simulink library "hcu_lib"  (Simulink 7.4)
settings: Solver=ode45  SolverMode=SingleTasking  StartTime=0.0  StopTime=10.0  RelTol=1e-3
undefined symbols (not defined in the file): FALSE, KPH2MPH, KPH2MPS, MPH2KPH, MPS2KPH, RADPS2RPM, RPM2RADPS, TRUE
libraries: hcu_lib x5, simulink x4
settings Model: Creator=gpf  LastModifiedBy=WX  ExtModeAutoUpdateStatusClock=off

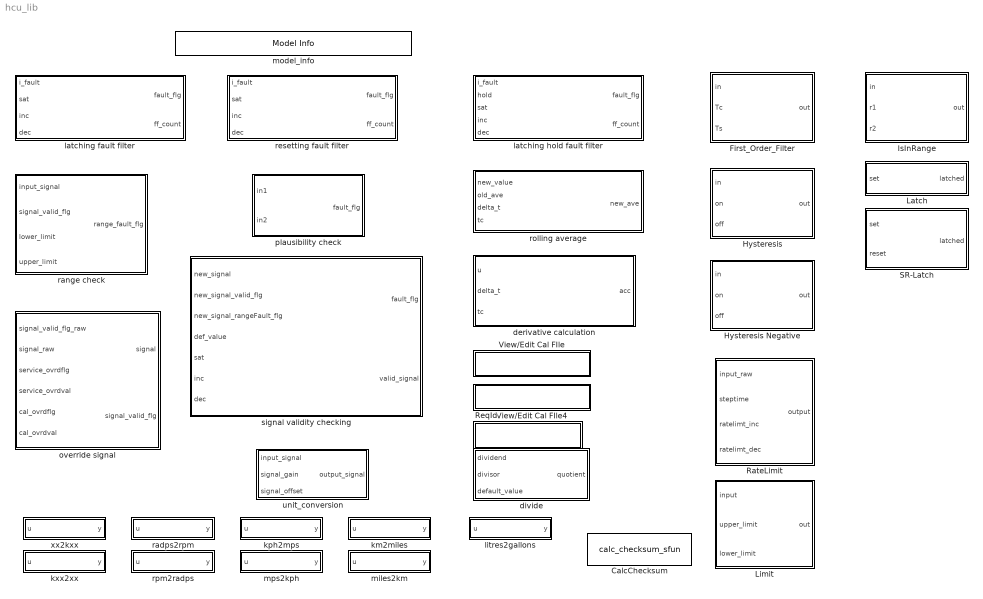
== system hcu_lib ==
  CalcChecksum : S-Function  FunctionName=calc_checksum_sfun  Parameters=seed_val  EnableBusSupport=off  mask(CalcChecksum){seed_val=40535}
      mask prompts: seed_val "seed (decimal)"
      mask help:
      | Sums the first 6 bytes on the input and returns a uint16 checksum value. The
      | input is a vector of 8 bytes (uint8).
      mask Display: fprintf('calc_checksum\nseed=%d',seed_val);
  First_Order_Filter : Subsystem  TreatAsAtomicUnit=on  RTWFileName=HCU_LIB
      settings: RTWFileNameOpts=User specified
  Hysteresis : Subsystem  TreatAsAtomicUnit=on  RTWFileName=HCU_LIB
      settings: RTWFileNameOpts=User specified
  Hysteresis Negative : Subsystem  TreatAsAtomicUnit=on  RTWFileName=HCU_LIB
      settings: RTWFileNameOpts=User specified
  IsInRange : Subsystem  TreatAsAtomicUnit=on  RTWFileName=HCU_LIB
      settings: RTWFileNameOpts=User specified
  Latch : Subsystem
  Limit : Subsystem  TreatAsAtomicUnit=on  RTWFileName=HCU_LIB
      settings: RTWFileNameOpts=User specified
  RateLimit : Subsystem  TreatAsAtomicUnit=on  RTWFileName=HCU_LIB
      settings: RTWFileNameOpts=User specified
  ReqId : Subsystem  mask(ReqId){req_str=HCU_000}
      mask prompts: req_str "Requirement:"
      mask help: Requirement Id
      mask Display: disp(sprintf('ReqId: %s',req_str));
  SR-Latch : Subsystem
  View/Edit Cal FIle : Subsystem  mask(edit){filename=foo}
      mask help:
      | Double-click to open the named file for viewing/editing.
      |
      | To set the name of the file opened, right-click on the block
      | and select Mask Parameters, and enter the name of the file,
      | which must be on the matlab path, without the .m extension.
      mask Help:
      | Double-click to open the named file for viewing/editing.
      | 
      | To set the name of the file opened, right-click on the block
      | and select Mask Parameters, and enter the name of the file,
      | which must be on the matlab path, without the .m extension.
      mask Display: disp(sprintf('Edit M-File: %s.m',filename));
  View/Edit Cal FIle4 : Subsystem  mask(run){filename=, run_on_load=off, run_on_init=off}
      mask prompts: run_on_load "run file on loading model"; run_on_init "run file on init"
      mask help:
      | Double-click to execute the named file.
      |
      | To set the name of the file, right-click on the block
      | and select Mask Parameters, and enter the name of the file,
      | which must be on the matlab path, without the .m extension.
      mask Help:
      | Double-click to execute the named file.
      | 
      | To set the name of the file, right-click on the block
      | and select Mask Parameters, and enter the name of the file,
      | which must be on the matlab path, without the .m extension.
      mask Display: disp(sprintf('Run M-File: %s.m',filename));
  derivative calculation : Subsystem  TreatAsAtomicUnit=on  RTWFileName=HCU_LIB  mask(Derative Block){lower_limit=, upper_limit=, time_const=}
      mask prompts: lower_limit "Lower Limit"; upper_limit "Upper Limit"; time_const "Time Constant"
      mask help: Derivative Calculation
      settings: RTWFileNameOpts=User specified
      mask Display: disp(['Derivative\nTC: ', get_param(gcb,'time_const'), '\nLower Limit: ', get_param(gcb, 'lower_limit'), '\nUpper Limit: ', get_param(gcb, 'upper_limit')])
  divide : Subsystem  TreatAsAtomicUnit=on  RTWFcnName=plaus_check
      settings: RTWSystemCode=Inline  RTWFcnNameOpts=User specified
      mask Type: divide
      mask Description: Performs a division operation. If the divisor is found to be between -0.00001 and +0.00001 then a failsafe value is passed to the output.
      mask Display: disp('Divide');
  km2miles : Subsystem
      mask Type: Conversion
      mask Description: Convert kilometers to miles.
      mask Display: disp('km \rightarrow mile', 'texmode', 'on')
  kph2mps : Subsystem
      mask Type: Conversion
      mask Description: Convert Kilometers per hour to Meters per second
      mask Display: disp('km/h \rightarrow m/s', 'texmode', 'on')
  kxx2xx : Subsystem
      mask Type: Conversion
      mask Description: Multiply by 1000.
      mask Display: disp('kiloxx \rightarrow xx', 'texmode', 'on')
  latching fault filter : Subsystem  TreatAsAtomicUnit=on  RTWFcnName=ff_latching  RTWFileName=HCU_LIB
      settings: RTWFcnNameOpts=User specified  RTWFileNameOpts=User specified
      mask Type: Latching Fault Filter
      mask Description: Fault filter block - Latches the fault output flag to TRUE if the input flag is repeatedly set True.
      mask Display: disp('Latching\nFault Filter')
  latching hold fault filter : Subsystem  TreatAsAtomicUnit=on  RTWFcnName=ff_latchhold  RTWFileName=HCU_LIB  mask(Latching Holdable Fault Filter){inc=, dec=, sat=}
      mask prompts: inc "increment"; dec "decrement"; sat "limit"
      mask help: Fault Filter Block - Latches output flag once set. Also fault count can be held at a value if the hold input is set.
      settings: RTWFcnNameOpts=User specified  RTWFileNameOpts=User specified
      mask Display: disp('Latching Holdable\nFault Filter')
  litres2gallons : Subsystem  mask(Conversion){UK=off}
      mask prompts: UK "UK Gallon"
      mask help: Convert litres to gallons.
      mask Display: disp('litre \rightarrow gallon', 'texmode', 'on')
  miles2km : Subsystem
      mask Type: Conversion
      mask Description: Convert kilometers to miles.
      mask Display: disp('mile \rightarrow km', 'texmode', 'on')
  model_info : simulink/Model-Wide Utilities/Model Info  SystemSampleTime=-1  InitialBlockCM=None  BlockCM=None  Frame=on  DisplayStringWithTags=$Id: hcu_lib.mdl 10 2009-03-27 10:09:46Z pgilhead $  HorizontalTextAlignment=Center  LeftAlignmentValue=0.5  SourceBlockDiagram=hcu_lib  TagMaxNumber=20
  mps2kph : Subsystem
      mask Type: Conversion
      mask Description: Convert Meters per second to Kilometers per hour
      mask Display: disp('m/s \rightarrow km/h', 'texmode', 'on')
  override signal : Subsystem  TreatAsAtomicUnit=on  RTWFcnName=srvc_ovrd  RTWFileName=HCU_LIB
      settings: RTWSystemCode=Inline  RTWFcnNameOpts=User specified  RTWFileNameOpts=User specified
      mask Type: override signal
      mask Description: Block facilitates the override of a raw input signal by another value, either from a service tool or from a calibration tool. Outputting signal valid flag from raw input except outputting signal valid flag as Valid if service tool or calibration value is used
  plausibility check : Subsystem  TreatAsAtomicUnit=on  RTWFcnName=plaus_check  RTWFileName=HCU_LIB  mask(Plausibility Check){limit=}
      mask prompts: limit "Comparison Limit"
      mask help: Plausibilty Check Block - compares the absolute difference between inputs and checks if within calibrated limit [ 0 - within limit ; 1 - greater than limit]
      settings: RTWFcnNameOpts=User specified  RTWFileNameOpts=User specified
      mask Display: disp(['Plausibility\nCheck\nLimit: ' get_param(gcb,'limit')])
  radps2rpm : Subsystem
      mask Description: Converst radians per second to revolutions per minute.
      mask Display: disp('rad/s \rightarrow rpm', 'texmode', 'on')
  range check : Subsystem  TreatAsAtomicUnit=on  RTWFcnName=range_check  RTWFileName=HCU_LIB
      settings: RTWFcnNameOpts=User specified  RTWFileNameOpts=User specified
      mask Type: Range Check
      mask Description: Performs a range check of the input signal against a defined acceptable signal range.  Outside of the defined range, an instantaneous fault flag will be set true.
      mask Display: disp('RC')
  resetting fault filter : Subsystem  TreatAsAtomicUnit=on  RTWFcnName=ff_resetting  RTWFileName=HCU_LIB
      settings: RTWFcnNameOpts=User specified  RTWFileNameOpts=User specified
      mask Type: Resetting Fault Filter
      mask Description: Fault Filter block - Will reset output fault flag after a Calibratable number of faultless inputs.
      mask Display: disp('Resetting\nFault Filter')
  rolling average : Subsystem  TreatAsAtomicUnit=on  RTWFcnName=rolav_tc  RTWFileName=HCU_LIB  mask(Rolling Average){}
      mask help:
      | Rolling Average - Time Constant.  This filter block is the first order approximation using a time constant.  Inputs include the time constant (entered through this dialogue), old_ave which is the previous average value, new_value which is the new filter to filter toward.
      |
      | The sample_interval which is elapsed time over which to perform the filter equation is computed internally - THIS BLOCK MUST BE CALLED EACH PASS to work as expected.
      settings: RTWFcnNameOpts=User specified  RTWFileNameOpts=User specified
      mask Display: disp('Rolling Average - TC')
  rpm2radps : Subsystem
      mask Description: Converts radians per second to revolutions per minute.
      mask Display: disp('rpm \rightarrow rad/s', 'texmode', 'on')
  signal validity checking : Subsystem  TreatAsAtomicUnit=on  RTWFcnName=sig_valid_check  RTWFileName=HCU_LIB
      settings: RTWFcnNameOpts=User specified  RTWFileNameOpts=User specified
      mask Type: signal validity checking
      mask Description: Block checks that the input signal is both in range and available. If either is not the case the block will temporarily output the last valid value or, after confirming a longer term fault, will output a default value (Calibratable). If the input signal continues to be faulty the fault flag output will be set after a calibratable number of failing values.
  unit_conversion : Subsystem  TreatAsAtomicUnit=on  RTWFcnName=unit_conversion
      settings: RTWSystemCode=Inline  RTWFcnNameOpts=User specified
      mask Description: Unit Conversion
  xx2kxx : Subsystem
      mask Type: Conversion
      mask Description: Divides by 1000.
      mask Display: disp('xx \rightarrow kiloxx', 'texmode', 'on')

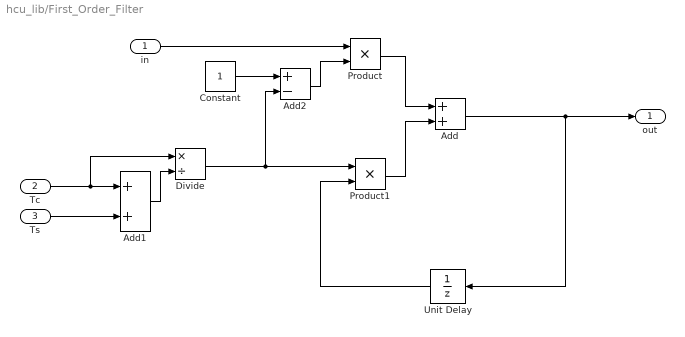
== system hcu_lib/First_Order_Filter ==
  in : Inport
  Tc : Inport  Port=2
  Ts : Inport  Port=3
  Add : Sum  OutDataType=fixdt(1, 16)  OutScaling=2^-10
  Add1 : Sum  OutDataType=fixdt(1, 16)  OutScaling=2^-10
  Add2 : Sum  Inputs=+-  OutDataType=fixdt(1, 16)  OutScaling=2^-10
  Constant : Constant  OutDataTypeMode=single  OutDataType=fixdt(1, 16)  OutScaling=2^0  OutDataTypeStr=single
  Divide : Product  Inputs=*/  OutDataType=fixdt(1, 16)  OutScaling=2^-10
  Product : Product  OutDataType=fixdt(1, 16)  OutScaling=2^0  RndMeth=Zero
  Product1 : Product  OutDataType=fixdt(1, 16)  OutScaling=2^0  RndMeth=Zero
  Unit Delay : UnitDelay  SampleTime=-1
  out : Outport
  wires:
  Unit Delay/1 -> Product1/2
  Tc/1 -> Add1/1, Divide/1
  Ts/1 -> Add1/2
  Add1/1 -> Divide/2
  Constant/1 -> Add2/1
  Divide/1 -> Add2/2, Product1/1
  in/1 -> Product/1
  Add2/1 -> Product/2
  Product/1 -> Add/1
  Product1/1 -> Add/2
  Add/1 -> out/1, Unit Delay/1

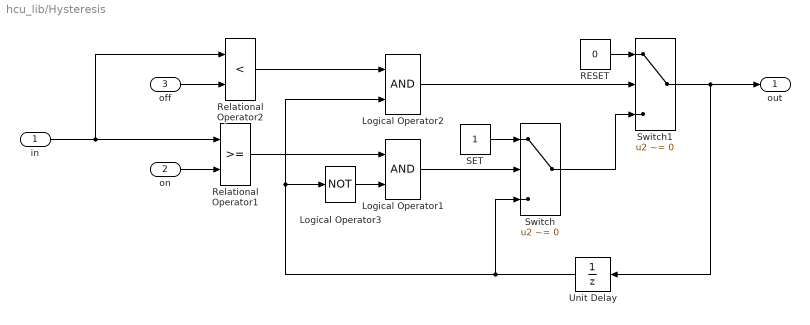
== system hcu_lib/Hysteresis ==
  in : Inport
  on : Inport  Port=2
  off : Inport  Port=3
  Logical Operator1 : Logic  AllPortsSameDT=off  OutDataTypeMode=boolean  LogicDataType=fixdt(0, 8)  OutDataTypeStr=boolean
  Logical Operator2 : Logic  AllPortsSameDT=off  OutDataTypeMode=boolean  LogicDataType=fixdt(0, 8)  OutDataTypeStr=boolean
  Logical Operator3 : Logic  Operator=NOT  AllPortsSameDT=off  OutDataTypeMode=boolean  LogicDataType=fixdt(0, 8)  OutDataTypeStr=boolean
  RESET : Constant  Value=0  OutDataTypeMode=boolean  OutDataType=fixdt(1, 16)  OutScaling=2^0  OutDataTypeStr=boolean
  Relational Operator1 : RelationalOperator  LogicOutDataTypeMode=boolean  LogicDataType=fixdt(0, 8)  OutDataTypeStr=boolean
  Relational Operator2 : RelationalOperator  Operator=<  LogicOutDataTypeMode=boolean  LogicDataType=fixdt(0, 8)  OutDataTypeStr=boolean
  SET : Constant  OutDataTypeMode=boolean  OutDataType=fixdt(1, 16)  OutScaling=2^0  OutDataTypeStr=boolean
  Switch : Switch  Criteria=u2 ~= 0  OutDataType=fixdt(1, 16)  OutScaling=2^0
  Switch1 : Switch  Criteria=u2 ~= 0  OutDataType=fixdt(1, 16)  OutScaling=2^0
  Unit Delay : UnitDelay  SampleTime=-1
  out : Outport
  wires:
  in/1 -> Relational Operator1/1, Relational Operator2/1
  on/1 -> Relational Operator1/2
  off/1 -> Relational Operator2/2
  Relational Operator1/1 -> Logical Operator1/1
  Relational Operator2/1 -> Logical Operator2/1
  Logical Operator1/1 -> Switch/2
  SET/1 -> Switch/1
  Switch/1 -> Switch1/3
  Logical Operator2/1 -> Switch1/2
  RESET/1 -> Switch1/1
  Switch1/1 -> out/1, Unit Delay/1
  Unit Delay/1 -> Switch/3, Logical Operator3/1, Logical Operator2/2
  Logical Operator3/1 -> Logical Operator1/2

== system hcu_lib/Hysteresis Negative ==
  in : Inport
  on : Inport  Port=2
  off : Inport  Port=3
  Hysteresis : hcu_lib/Hysteresis  SystemSampleTime=-1
  Logical Operator3 : Logic  Operator=NOT  AllPortsSameDT=off  OutDataTypeMode=boolean  LogicDataType=fixdt(0, 8)  OutDataTypeStr=boolean
  out : Outport
  wires:
  Hysteresis/1 -> Logical Operator3/1
  in/1 -> Hysteresis/1
  Logical Operator3/1 -> out/1
  off/1 -> Hysteresis/2
  on/1 -> Hysteresis/3

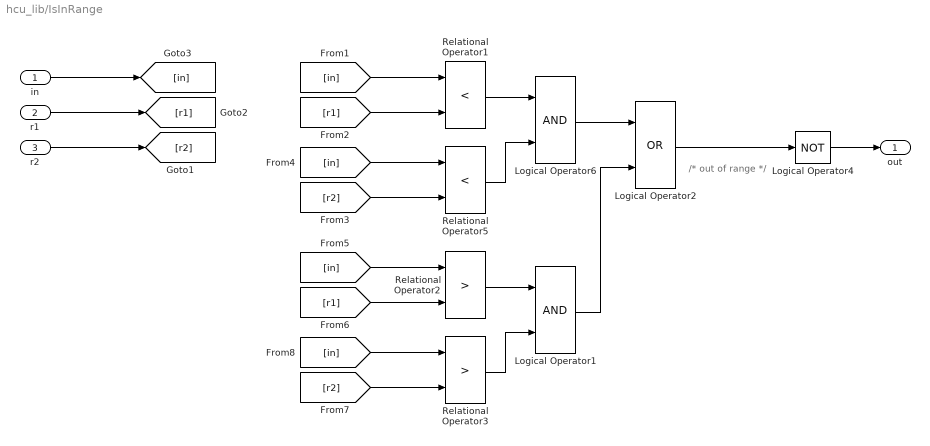
== system hcu_lib/IsInRange ==
  note: /* out of range */
  in : Inport
  r1 : Inport  Port=2
  r2 : Inport  Port=3
  Logical Operator1 : Logic  AllPortsSameDT=off  OutDataTypeMode=boolean  LogicDataType=fixdt(0, 8)  OutDataTypeStr=boolean
  Logical Operator2 : Logic  Operator=OR  AllPortsSameDT=off  OutDataTypeMode=boolean  LogicDataType=fixdt(0, 8)  OutDataTypeStr=boolean
  Logical Operator4 : Logic  Operator=NOT  AllPortsSameDT=off  OutDataTypeMode=boolean  LogicDataType=fixdt(0, 8)  OutDataTypeStr=boolean
  Logical Operator6 : Logic  AllPortsSameDT=off  OutDataTypeMode=boolean  LogicDataType=fixdt(0, 8)  OutDataTypeStr=boolean
  Relational Operator1 : RelationalOperator  Operator=<  LogicOutDataTypeMode=boolean  LogicDataType=fixdt(0, 8)  OutDataTypeStr=boolean
  Relational Operator2 : RelationalOperator  Operator=>  LogicOutDataTypeMode=boolean  LogicDataType=fixdt(0, 8)  OutDataTypeStr=boolean
  Relational Operator3 : RelationalOperator  Operator=>  LogicOutDataTypeMode=boolean  LogicDataType=fixdt(0, 8)  OutDataTypeStr=boolean
  Relational Operator5 : RelationalOperator  Operator=<  LogicOutDataTypeMode=boolean  LogicDataType=fixdt(0, 8)  OutDataTypeStr=boolean
  out : Outport
  wires:
  Relational Operator1/1 -> Logical Operator6/1
  Relational Operator5/1 -> Logical Operator6/2
  Logical Operator6/1 -> Logical Operator2/1
  in/1 -> [in]
  r1/1 -> [r1]
  r2/1 -> [r2]
  [in] -> Relational Operator1/1
  [r1] -> Relational Operator1/2
  [in] -> Relational Operator5/1
  [r2] -> Relational Operator5/2
  Relational Operator2/1 -> Logical Operator1/1
  Relational Operator3/1 -> Logical Operator1/2
  [in] -> Relational Operator2/1
  [r1] -> Relational Operator2/2
  [in] -> Relational Operator3/1
  [r2] -> Relational Operator3/2
  Logical Operator1/1 -> Logical Operator2/2
  Logical Operator2/1 -> Logical Operator4/1
  Logical Operator4/1 -> out/1

== system hcu_lib/Latch ==
  set : Inport
  Switch1 : Switch  Criteria=u2 ~= 0  Threshold=0.5  OutDataType=fixdt(1, 16)  OutScaling=2^0
      settings: AttributesFormatString=<Criteria=%<Criteria>>
  Unit Delay : UnitDelay  SampleTime=-1
  latched : Outport
  wires:
  Unit Delay/1 -> Switch1/1, Switch1/2
  Switch1/1 -> Unit Delay/1, latched/1
  set/1 -> Switch1/3

== system hcu_lib/Limit ==
  input : Inport
  upper_limit : Inport  Port=2
  lower_limit : Inport  Port=3
  MinMax10 : MinMax  Function=max  Inputs=2  OutDataType=fixdt(1, 16)  OutScaling=2^0
  MinMax5 : MinMax  Inputs=2  OutDataType=fixdt(1, 16)  OutScaling=2^0
  out : Outport
  wires:
  lower_limit/1 -> MinMax10/2
  upper_limit/1 -> MinMax5/2
  MinMax10/1 -> out/1
  input/1 -> MinMax5/1
  MinMax5/1 -> MinMax10/1

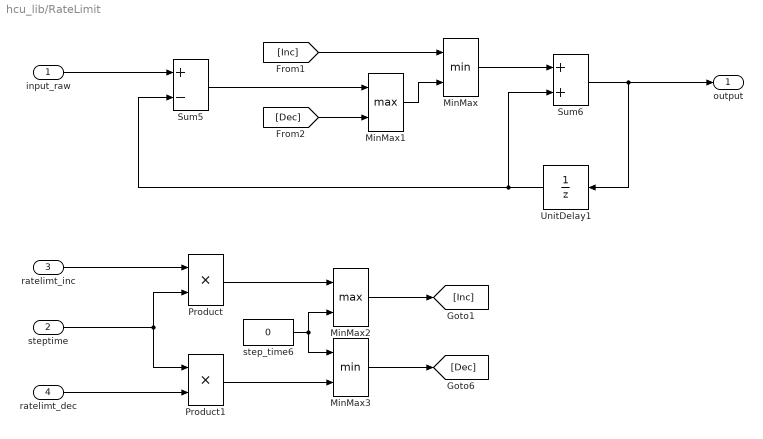
== system hcu_lib/RateLimit ==
  input_raw : Inport  OutDataType=sfix(16)  OutScaling=2^0
  steptime : Inport  Port=2  OutDataType=sfix(16)  OutScaling=2^0
  ratelimt_inc : Inport  Port=3  OutDataType=sfix(16)  OutScaling=2^0
  ratelimt_dec : Inport  Port=4  OutDataType=sfix(16)  OutScaling=2^0
  MinMax : MinMax  Inputs=2  OutDataType=sfix(16)  OutScaling=2^0
  MinMax1 : MinMax  Function=max  Inputs=2  OutDataType=sfix(16)  OutScaling=2^0
  MinMax2 : MinMax  Function=max  Inputs=2  OutDataType=sfix(16)  OutScaling=2^0
  MinMax3 : MinMax  Inputs=2  OutDataType=sfix(16)  OutScaling=2^0
  Product : Product  OutDataType=sfix(16)  OutScaling=2^0  RndMeth=Zero
  Product1 : Product  OutDataType=sfix(16)  OutScaling=2^0  RndMeth=Zero
  Sum5 : Sum  Inputs=+-  OutDataType=sfix(16)  OutScaling=2^0
  Sum6 : Sum  OutDataType=sfix(16)  OutScaling=2^0
  UnitDelay1 : UnitDelay  SampleTime=-1
  step_time6 : Constant  Value=0  OutDataTypeMode=single  OutDataType=sfix(16)  OutScaling=2^0  OutDataTypeStr=single
  output : Outport
  wires:
  ratelimt_dec/1 -> Product1/2
  steptime/1 -> Product1/1, Product/2
  Sum5/1 -> MinMax1/1
  [Dec] -> MinMax1/2
  [Inc] -> MinMax/1
  MinMax1/1 -> MinMax/2
  MinMax/1 -> Sum6/1
  input_raw/1 -> Sum5/1
  Sum6/1 -> output/1, UnitDelay1/1
  UnitDelay1/1 -> Sum5/2, Sum6/2
  Product/1 -> MinMax2/1
  Product1/1 -> MinMax3/2
  step_time6/1 -> MinMax2/2, MinMax3/1
  MinMax2/1 -> [Inc]
  MinMax3/1 -> [Dec]
  ratelimt_inc/1 -> Product/1

== system hcu_lib/ReqId ==

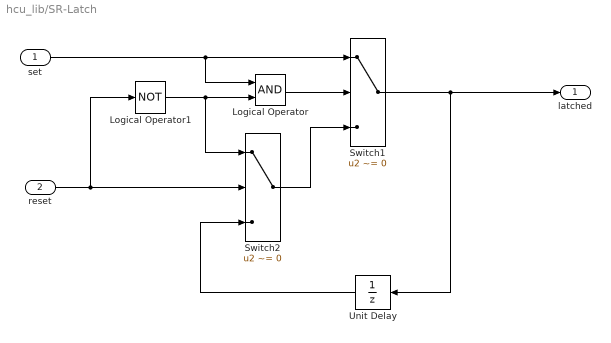
== system hcu_lib/SR-Latch ==
  set : Inport
  reset : Inport  Port=2
  Logical Operator : Logic  AllPortsSameDT=off  OutDataTypeMode=boolean  LogicDataType=fixdt(0, 8)  OutDataTypeStr=boolean
  Logical Operator1 : Logic  Operator=NOT  AllPortsSameDT=off  OutDataTypeMode=boolean  LogicDataType=fixdt(0, 8)  OutDataTypeStr=boolean
  Switch1 : Switch  Criteria=u2 ~= 0  Threshold=0.5  OutDataType=fixdt(1, 16)  OutScaling=2^0
      settings: AttributesFormatString=<Criteria=%<Criteria>>
  Switch2 : Switch  Criteria=u2 ~= 0  Threshold=0.5  OutDataType=fixdt(1, 16)  OutScaling=2^0
      settings: AttributesFormatString=<Criteria=%<Criteria>>
  Unit Delay : UnitDelay  SampleTime=-1
  latched : Outport
  wires:
  Logical Operator1/1 -> Switch2/1, Logical Operator/2
  Logical Operator/1 -> Switch1/2
  Switch2/1 -> Switch1/3
  Unit Delay/1 -> Switch2/3
  reset/1 -> Logical Operator1/1, Switch2/2
  set/1 -> Logical Operator/1, Switch1/1
  Switch1/1 -> latched/1, Unit Delay/1

== system hcu_lib/View/Edit Cal FIle ==

== system hcu_lib/View/Edit Cal FIle4 ==

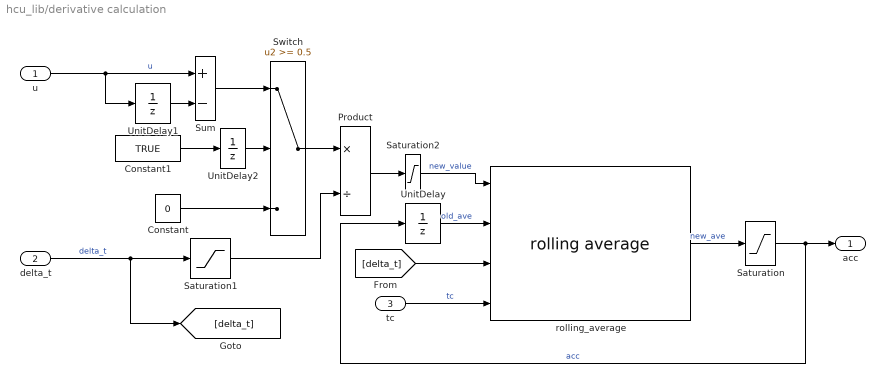
== system hcu_lib/derivative calculation ==
  u : Inport  OutDataType=sfix(16)  OutScaling=2^0
  delta_t : Inport  Port=2  OutDataType=sfix(16)  OutScaling=2^0
  tc : Inport  Port=3  OutDataType=sfix(16)  OutScaling=2^0
  Constant : Constant  Tag=struct('comment',struct('text','','placement',1),'output',struct('width',1,'name','$S_$B','unit','','type','Int16','offset',0,'max',NaN,'min',NaN,'freeze',1,'lsb',1,'arb',0,'class','default','address','','description','','value','0','tolerance',1,'show',0),'date',731450.689904282)  Value=0  OutDataType=sfix(16)  OutScaling=2^0
  Constant1 : Constant  Tag=struct('comment',struct('text','','placement',1),'output',struct('width',1,'name','$S_$B','unit','','type','Int16','offset',0,'max',NaN,'min',NaN,'freeze',1,'lsb',1,'arb',0,'class','default','address','','description','','value','2','tolerance',1,'show',0),'date',731450.690075)  Value=TRUE  OutDataType=sfix(16)  OutScaling=2^0
  Product : Product  Tag=struct('comment',struct('text','','placement',1),'logdata',struct('maxnumvals',inf,'plotchannels',[],'stepsize',0,'downsampling',1,'loggingmode',3,'channels',1),'output',struct('width',1,'name','$S_$B','unit','','type','Int32Bin15','offset',0,'max',65535,'min',-65536,'freeze',1,'lsb',2^-15,'arb',0,'class','default','address','','description','','autoscalingmode',1,'lowerheadroom',1,'upperheadroom',1,'headroomunit','bit','checkmin',0,'checkmax',0,'show',0),'inputs','*/','exceptionhandling',1,'date',731458.438505301)  Inputs=*/  OutDataType=sfix(16)  OutScaling=2^0  SaturateOnIntegerOverflow=on  RndMeth=Zero  InputSameDT=on  OutDataTypeStr=Inherit: Same as first input
  Saturation : Saturate  UpperLimit=upper_limit  LowerLimit=lower_limit
  Saturation1 : Saturate  Tag=struct('comment',struct('text','','placement',1),'logdata',struct('maxnumvals',inf,'plotchannels',[],'stepsize',0,'downsampling',1,'loggingmode',3,'channels',1),'output',struct('width',1,'name','$S_$B','unit','s','type','Time16bin10','offset',0,'max',63.999,'min',0,'freeze',1,'lsb',2^-10,'arb',0,'class','default','address','','description','','autoscalingmode',1,'lowerheadroom',1,'upperheadroom',1,'headroomunit','bit','show',0),'lowerlimit',struct('width',1,'name','$S_$B_lower','unit','','type','Int16','offset',0,'max',NaN,'min',NaN,'freeze',1,'lsb',1,'arb',0,'class','default','address','','description','','value','12e-3','scalar',0),'upperlimit',struct('width',1,'name','$S_$B_upper','unit','','type','Int16','offset',0,'max',NaN,'min',NaN,'freeze',1,'lsb',1,'arb',0,'class','default','address','','description','','value','63.9','scalar',0),'date',731458.439118333)  UpperLimit=63.9  LowerLimit=12e-3
  Saturation2 : Saturate  Tag=struct('comment',struct('text','','placement',1),'logdata',struct('maxnumvals',inf,'plotchannels',[],'stepsize',0,'downsampling',1,'loggingmode',3,'channels',1),'output',struct('width',1,'name','$S_$B','unit','','type','Int32Bin15','offset',0,'max',65535,'min',-65536,'freeze',1,'lsb',2^-15,'arb',0,'class','default','address','','description','','autoscalingmode',1,'lowerheadroom',1,'upperheadroom',1,'headroomunit','bit','show',0),'lowerlimit',struct('width',1,'name','$S_$B_lower','unit','','type','Int16','offset',0,'max',NaN,'min',NaN,'freeze',1,'lsb',1,'arb',0,'class','default','address','','description','','value','-65536','scalar',0),'upperlimit',struct('width',1,'name','$S_$B_upper','unit','','type','Int16','offset',0,'max',NaN,'min',NaN,'freeze',1,'lsb',1,'arb',0,'class','default','address','','description','','value','65535','scalar',0),'date',731455.58891853)  UpperLimit=65535  LowerLimit=-65536
  Sum : Sum  Tag=struct('comment',struct('text','','placement',1),'logdata',struct('maxnumvals',inf,'plotchannels',[],'stepsize',0,'downsampling',1,'loggingmode',3,'channels',1),'output',struct('width',1,'name','$S_$B','unit','','type','Int32Bin15','offset',0,'max',65535,'min',-65536,'freeze',1,'lsb',2^-15,'arb',0,'class','default','address','','description','','autoscalingmode',1,'lowerheadroom',1,'upperheadroom',1,'headroomunit','bit','checkmin',0,'checkmax',0,'show',0),'inputs','+-','date',731450.688943275)  Inputs=+-  OutDataType=sfix(16)  OutScaling=2^0  SaturateOnIntegerOverflow=on  InputSameDT=on  OutDataTypeStr=Inherit: Same as first input
  Switch : Switch  Tag=struct('comment',struct('text','','placement',1),'logdata',struct('maxnumvals',inf,'plotchannels',[],'stepsize',0,'downsampling',1,'loggingmode',3,'channels',1),'output',struct('width',1,'name','$S_$B','unit','','type','Int32Bin15','offset',0,'max',65535,'min',-65536,'freeze',1,'lsb',2^-15,'arb',0,'class','default','address','','description','','autoscalingmode',1,'lowerheadroom',1,'upperheadroom',1,'headroomunit','bit','checkmin',0,'checkmax',0,'show',0),'threshold',struct('width',1,'name','$S_$B_threshold','unit','','type','Int16','offset',0,'max',NaN,'min',NaN,'freeze',1,'lsb',1,'arb',0,'class','default','address','','description','','value','1','scalar',0),'date',731458.438569977)  Threshold=0.5  SaturateOnIntegerOverflow=on  InputSameDT=on
  UnitDelay : UnitDelay  Tag=struct('comment',struct('text','','placement',1),'logdata',struct('maxnumvals',inf,'plotchannels',[],'stepsize',0,'downsampling',1,'loggingmode',3,'channels',1),'output',struct('width',1,'name','$S_$B','unit','','type','Int32Bin15','offset',0,'max',65535,'min',-65536,'freeze',1,'lsb',2^-15,'arb',0,'class','default','address','','description','','autoscalingmode',1,'lowerheadroom',1,'upperheadroom',1,'headroomunit','bit','checkmin',0,'checkmax',0,'show',0,'initial','0'),'state',0,'dt','-1','date',731638.587904039)  SampleTime=-1
  UnitDelay1 : UnitDelay  Tag=struct('comment',struct('text','','placement',1),'logdata',struct('maxnumvals',inf,'plotchannels',[],'stepsize',0,'downsampling',1,'loggingmode',3,'channels',1),'output',struct('width',1,'name','$S_$B','unit','','type','Int32Bin15','offset',0,'max',65535,'min',-65536,'freeze',1,'lsb',2^-15,'arb',0,'class','default','address','','description','','autoscalingmode',1,'lowerheadroom',1,'upperheadroom',1,'headroomunit','bit','checkmin',0,'checkmax',0,'show',0,'initial','0'),'state',0,'dt','-1','date',731450.687911019)  SampleTime=-1
  UnitDelay2 : UnitDelay  Tag=struct('comment',struct('text','','placement',1),'logdata',struct('maxnumvals',inf,'plotchannels',[],'stepsize',0,'downsampling',1,'loggingmode',3,'channels',1),'output',struct('width',1,'name','$S_$B','unit','','type','UInt8','offset',0,'max',255,'min',0,'freeze',1,'lsb',1,'arb',0,'class','default','address','','description','','autoscalingmode',1,'lowerheadroom',1,'upperheadroom',1,'headroomunit','bit','checkmin',0,'checkmax',0,'show',0,'initial','0'),'state',0,'dt','-1','date',731450.690382801)  X0=FALSE  SampleTime=-1  StateIdentifier=first_pass
  rolling_average : hcu_lib/rolling average  SystemSampleTime=-1
  acc : Outport  OutDataType=sfix(16)  OutScaling=2^0
  wires:
  Saturation/1 -> UnitDelay/1, acc/1  "acc"
  rolling_average/1 -> Saturation/1  "new_ave"
  UnitDelay/1 -> rolling_average/2  "old_ave"
  u/1 -> Sum/1, UnitDelay1/1  "u"
  UnitDelay1/1 -> Sum/2
  Product/1 -> Saturation2/1
  Sum/1 -> Switch/1
  delta_t/1 -> Saturation1/1, [delta_t]  "delta_t"
  Switch/1 -> Product/1
  Constant/1 -> Switch/3
  UnitDelay2/1 -> Switch/2
  Constant1/1 -> UnitDelay2/1
  Saturation1/1 -> Product/2
  Saturation2/1 -> rolling_average/1  "new_value"
  [delta_t] -> rolling_average/3
  tc/1 -> rolling_average/4  "tc"

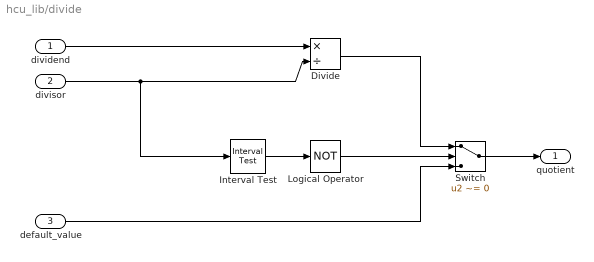
== system hcu_lib/divide ==
  dividend : Inport  OutDataType=sfix(16)  OutScaling=2^0
  divisor : Inport  Port=2  OutDataType=sfix(16)  OutScaling=2^0
  default_value : Inport  Port=3  OutDataType=sfix(16)  OutScaling=2^0
  Divide : Product  Inputs=*/  OutDataType=sfix(16)  OutScaling=2^-10
  Interval Test : simulink/Logic and Bit Operations/Interval Test  SystemSampleTime=-1  IntervalClosedRight=on  uplimit=single(0.00001)  IntervalClosedLeft=on  lowlimit=single(-0.00001)  LogicOutDataTypeMode=boolean
  Logical Operator : Logic  Operator=NOT  AllPortsSameDT=off  OutDataTypeMode=boolean  OutDataTypeStr=boolean
  Switch : Switch  Criteria=u2 ~= 0  OutDataType=sfix(16)  OutScaling=2^0
  quotient : Outport  OutDataType=sfix(16)  OutScaling=2^0
  wires:
  dividend/1 -> Divide/1
  divisor/1 -> Divide/2, Interval Test/1
  Divide/1 -> Switch/1
  Switch/1 -> quotient/1
  Interval Test/1 -> Logical Operator/1
  default_value/1 -> Switch/3
  Logical Operator/1 -> Switch/2

== system hcu_lib/km2miles ==
  u : Inport  OutDataType=sfix(16)  OutScaling=2^0
  Gain : Gain  Gain=KPH2MPH  ParameterDataType=sfix(16)  ParameterScaling=2^0  OutDataType=sfix(16)  OutScaling=2^0
  y : Outport  OutDataType=sfix(16)  OutScaling=2^0
  wires:
  Gain/1 -> y/1  "y"
  u/1 -> Gain/1  "u"

== system hcu_lib/kph2mps ==
  u : Inport  OutDataType=sfix(16)  OutScaling=2^0
  Gain : Gain  Gain=KPH2MPS  ParameterDataType=sfix(16)  ParameterScaling=2^0  OutDataType=sfix(16)  OutScaling=2^0
  y : Outport  OutDataType=sfix(16)  OutScaling=2^0
  wires:
  Gain/1 -> y/1  "y"
  u/1 -> Gain/1  "u"

== system hcu_lib/kxx2xx ==
  u : Inport  OutDataType=sfix(16)  OutScaling=2^0
  Gain : Gain  Gain=1000  ParameterDataType=sfix(16)  ParameterScaling=2^0  OutDataType=sfix(16)  OutScaling=2^0
  y : Outport  OutDataType=sfix(16)  OutScaling=2^0
  wires:
  u/1 -> Gain/1  "u"
  Gain/1 -> y/1  "y"

== system hcu_lib/latching fault filter ==
  i_fault : Inport  OutDataType=sfix(16)  OutScaling=2^0
  sat : Inport  Port=2  OutDataType=sfix(16)  OutScaling=2^0
  inc : Inport  Port=3  OutDataType=sfix(16)  OutScaling=2^0
  dec : Inport  Port=4  OutDataType=sfix(16)  OutScaling=2^0
  lff_ctl : Stateflow chart
  fault_flg : Outport  OutDataType=sfix(16)  OutScaling=2^0
  ff_count : Outport  Port=2  OutDataType=sfix(16)  OutScaling=2^0
  wires:
  dec/1 -> lff_ctl/3(dec)  "dec"
  i_fault/1 -> lff_ctl/4(i_fault)  "i_fault"
  lff_ctl/1(fault_flg) -> fault_flg/1  "fault_flg"
  inc/1 -> lff_ctl/2(inc)  "inc"
  sat/1 -> lff_ctl/1(sat)  "sat"
  lff_ctl/2(ff_count) -> ff_count/1  "ff_count"

== system hcu_lib/latching hold fault filter ==
  i_fault : Inport  OutDataType=sfix(16)  OutScaling=2^0
  hold : Inport  Port=2  OutDataType=sfix(16)  OutScaling=2^0
  sat : Inport  Port=3  OutDataType=sfix(16)  OutScaling=2^0
  inc : Inport  Port=4  OutDataType=sfix(16)  OutScaling=2^0
  dec : Inport  Port=5  OutDataType=sfix(16)  OutScaling=2^0
  lhff_ctl : Stateflow chart
  fault_flg : Outport  OutDataType=sfix(16)  OutScaling=2^0
  ff_count : Outport  Port=2  OutDataType=sfix(16)  OutScaling=2^0
  wires:
  dec/1 -> lhff_ctl/3(dec)  "inc"
  hold/1 -> lhff_ctl/5(hold)  "hold"
  i_fault/1 -> lhff_ctl/4(i_fault)  "i_fault"
  lhff_ctl/1(fault_flg) -> fault_flg/1  "fault_flg"
  inc/1 -> lhff_ctl/2(inc)  "inc"
  sat/1 -> lhff_ctl/1(sat)  "sat"
  lhff_ctl/2(ff_count) -> ff_count/1  "ff_count"

== system hcu_lib/litres2gallons ==
  u : Inport  OutDataType=sfix(16)  OutScaling=2^0
  Constant : Constant  Value=UK  OutDataTypeMode=boolean  OutDataType=sfix(16)  OutScaling=2^0  OutDataTypeStr=boolean
  Switch : Switch  Threshold=0.5  ZeroCross=off
  UK : Gain  Gain=0.2199692483  ParameterDataType=sfix(16)  ParameterScaling=2^0  OutDataType=sfix(16)  OutScaling=2^0
  US : Gain  Gain=0.2641720524  ParameterDataType=sfix(16)  ParameterScaling=2^0  OutDataType=sfix(16)  OutScaling=2^0
  y : Outport  OutDataType=sfix(16)  OutScaling=2^0
  wires:
  UK/1 -> Switch/1
  US/1 -> Switch/3
  u/1 -> UK/1, US/1  "u"
  Switch/1 -> y/1  "y"
  Constant/1 -> Switch/2

== system hcu_lib/miles2km ==
  u : Inport  OutDataType=sfix(16)  OutScaling=2^0
  Gain : Gain  Gain=MPH2KPH  ParameterDataType=sfix(16)  ParameterScaling=2^0  OutDataType=sfix(16)  OutScaling=2^0
  y : Outport  OutDataType=sfix(16)  OutScaling=2^0
  wires:
  u/1 -> Gain/1  "u"
  Gain/1 -> y/1  "y"

== system hcu_lib/mps2kph ==
  u : Inport  OutDataType=sfix(16)  OutScaling=2^0
  Gain : Gain  Gain=MPS2KPH  ParameterDataType=sfix(16)  ParameterScaling=2^0  OutDataType=sfix(16)  OutScaling=2^0
  y : Outport  OutDataType=sfix(16)  OutScaling=2^0
  wires:
  u/1 -> Gain/1  "u"
  Gain/1 -> y/1  "y"

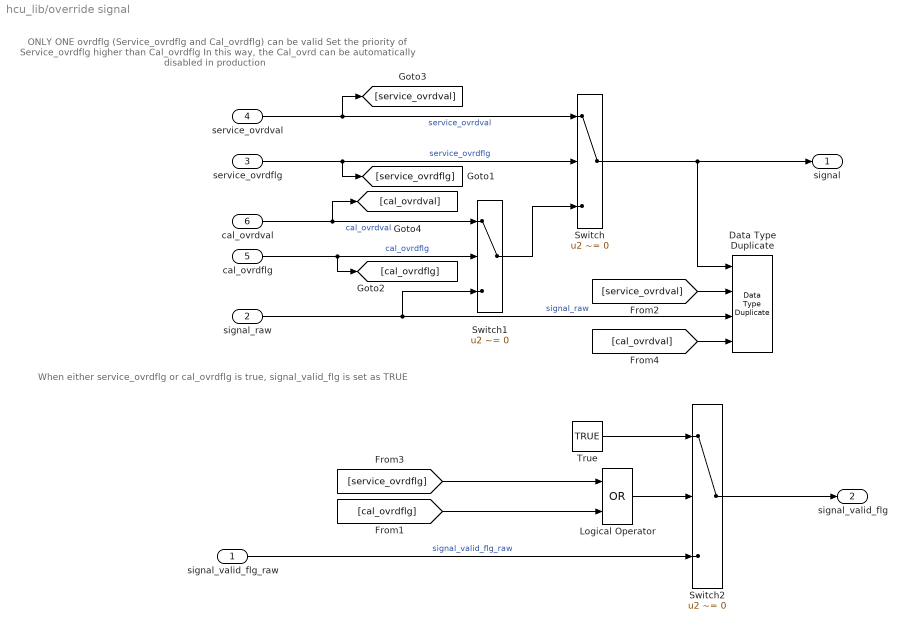
== system hcu_lib/override signal ==
  note: When either service_ovrdflg or cal_ovrdflg is true, signal_valid_flg is set as TRUE
  note: ONLY ONE ovrdflg (Service_ovrdflg and Cal_ovrdflg) can be valid
      | Set the priority of Service_ovrdflg higher than Cal_ovrdflg
      | In this way, the Cal_ovrd can be automatically disabled in production
  signal_valid_flg_raw : Inport
  signal_raw : Inport  Port=2
  service_ovrdflg : Inport  Port=3
  service_ovrdval : Inport  Port=4
  cal_ovrdflg : Inport  Port=5
  cal_ovrdval : Inport  Port=6
  Data Type Duplicate : simulink/Signal Attributes/Data Type Duplicate  NumInputPorts=4
  Logical Operator : Logic  Operator=OR  AllPortsSameDT=off  OutDataTypeMode=boolean  OutDataTypeStr=boolean
  Switch : Switch  Criteria=u2 ~= 0  Threshold=0.5  OutDataType=sfix(16)  OutScaling=2^0
  Switch1 : Switch  Criteria=u2 ~= 0  Threshold=0.5  OutDataType=sfix(16)  OutScaling=2^0
  Switch2 : Switch  Criteria=u2 ~= 0  Threshold=0.5  OutDataType=sfix(16)  OutScaling=2^0
  True : Constant  Value=TRUE  OutDataTypeMode=boolean  OutDataType=sfix(16)  OutScaling=2^0  OutDataTypeStr=boolean
  signal : Outport
  signal_valid_flg : Outport  Port=2
  wires:
  signal_valid_flg_raw/1 -> Switch2/3  "signal_valid_flg_raw"
  Switch2/1 -> signal_valid_flg/1
  True/1 -> Switch2/1
  Logical Operator/1 -> Switch2/2
  Switch1/1 -> Switch/3
  signal_raw/1 -> Switch1/3, Data Type Duplicate/3  "signal_raw"
  cal_ovrdval/1 -> Switch1/1, [cal_ovrdval]  "cal_ovrdval"
  service_ovrdval/1 -> Switch/1, [service_ovrdval]  "service_ovrdval"
  cal_ovrdflg/1 -> Switch1/2, [cal_ovrdflg]  "cal_ovrdflg"
  service_ovrdflg/1 -> Switch/2, [service_ovrdflg]  "service_ovrdflg"
  Switch/1 -> signal/1, Data Type Duplicate/1
  [service_ovrdflg] -> Logical Operator/1
  [cal_ovrdflg] -> Logical Operator/2
  [service_ovrdval] -> Data Type Duplicate/2
  [cal_ovrdval] -> Data Type Duplicate/4

== system hcu_lib/plausibility check ==
  in1 : Inport  OutDataType=sfix(16)  OutScaling=2^0
  in2 : Inport  Port=2  OutDataType=sfix(16)  OutScaling=2^0
  Abs : Abs  Tag=struct('comment',struct('text','','placement',1),'logdata',struct('maxnumvals',inf,'plotchannels',[],'stepsize',0,'downsampling',1,'loggingmode',3,'channels',1),'output',struct('width',1,'name','$S_$B','unit','','type','Int32Bin15','offset',0,'max',65535,'min',-65536,'freeze',1,'lsb',2^-15,'arb',0,'class','default','address','','description','','autoscalingmode',1,'lowerheadroom',1,'upperheadroom',1,'headroomunit','bit','checkmin',0,'checkmax',0,'show',0),'date',731458.540349433)  SaturateOnIntegerOverflow=on
  Constant : Constant  Value=limit  OutDataType=sfix(16)  OutScaling=2^0
  Relational Operator : RelationalOperator  Tag=struct('comment',struct('text','','placement',1),'logdata',struct('maxnumvals',inf,'plotchannels',[],'stepsize',0,'downsampling',1,'loggingmode',3,'channels',1),'operator','>','output',struct('class','default','type','Bool8','description','','address','','unit','','name','$S_$B'),'date',731458.540397882)  Operator=>  InputSameDT=on
  Sum : Sum  Tag=struct('comment',struct('text','','placement',1),'logdata',struct('maxnumvals',inf,'plotchannels',[],'stepsize',0,'downsampling',1,'loggingmode',3,'channels',1),'output',struct('width',1,'name','$S_$B','unit','','type','Int32Bin15','offset',0,'max',32767,'min',-32768,'freeze',1,'lsb',2^-16,'arb',0,'class','default','address','','description','','autoscalingmode',1,'lowerheadroom',1,'upperheadroom',1,'headroomunit','bit','checkmin',0,'checkmax',0,'show',0),'inputs','+-','date',731400.416541794)  Inputs=+-  OutDataType=sfix(16)  OutScaling=2^0  SaturateOnIntegerOverflow=on  InputSameDT=on  OutDataTypeStr=Inherit: Same as first input
  fault_flg : Outport  OutDataType=sfix(16)  OutScaling=2^0
  wires:
  Constant/1 -> Relational Operator/2
  Abs/1 -> Relational Operator/1
  Sum/1 -> Abs/1
  in1/1 -> Sum/1  "in1"
  in2/1 -> Sum/2  "in2"
  Relational Operator/1 -> fault_flg/1  "fault_flg"

== system hcu_lib/radps2rpm ==
  u : Inport  OutDataType=sfix(16)  OutScaling=2^0
  Gain : Gain  Gain=RADPS2RPM  ParameterDataType=sfix(16)  ParameterScaling=2^0  OutDataType=sfix(16)  OutScaling=2^0
  y : Outport  OutDataType=sfix(16)  OutScaling=2^0
  wires:
  u/1 -> Gain/1  "u"
  Gain/1 -> y/1  "y"

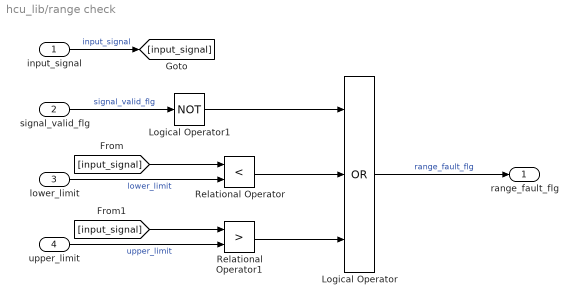
== system hcu_lib/range check ==
  input_signal : Inport  OutDataType=sfix(16)  OutScaling=2^0
  signal_valid_flg : Inport  Port=2  OutDataType=sfix(16)  OutScaling=2^0
  lower_limit : Inport  Port=3  OutDataType=sfix(16)  OutScaling=2^0
  upper_limit : Inport  Port=4  OutDataType=sfix(16)  OutScaling=2^0
  Logical Operator : Logic  Operator=OR  Inputs=3  AllPortsSameDT=off  OutDataTypeMode=boolean  OutDataTypeStr=boolean
  Logical Operator1 : Logic  Operator=NOT  AllPortsSameDT=off  OutDataTypeMode=boolean  OutDataTypeStr=boolean
  Relational Operator : RelationalOperator  Operator=<  LogicOutDataTypeMode=boolean  OutDataTypeStr=boolean
  Relational Operator1 : RelationalOperator  Operator=>  LogicOutDataTypeMode=boolean  OutDataTypeStr=boolean
  range_fault_flg : Outport  OutDataType=sfix(16)  OutScaling=2^0
  wires:
  Logical Operator/1 -> range_fault_flg/1  "range_fault_flg"
  input_signal/1 -> [input_signal]  "input_signal"
  signal_valid_flg/1 -> Logical Operator1/1  "signal_valid_flg"
  lower_limit/1 -> Relational Operator/2  "lower_limit"
  upper_limit/1 -> Relational Operator1/2  "upper_limit"
  Logical Operator1/1 -> Logical Operator/1
  [input_signal] -> Relational Operator/1
  Relational Operator/1 -> Logical Operator/2
  [input_signal] -> Relational Operator1/1
  Relational Operator1/1 -> Logical Operator/3

== system hcu_lib/resetting fault filter ==
  i_fault : Inport  OutDataType=sfix(16)  OutScaling=2^0
  sat : Inport  Port=2  OutDataType=sfix(16)  OutScaling=2^0
  inc : Inport  Port=3  OutDataType=sfix(16)  OutScaling=2^0
  dec : Inport  Port=4  OutDataType=sfix(16)  OutScaling=2^0
  rff_ctl : Stateflow chart
  fault_flg : Outport  OutDataType=sfix(16)  OutScaling=2^0
  ff_count : Outport  Port=2  OutDataType=sfix(16)  OutScaling=2^0
  wires:
  dec/1 -> rff_ctl/3(dec)  "dec"
  sat/1 -> rff_ctl/1(sat)  "sat"
  inc/1 -> rff_ctl/2(inc)  "inc"
  i_fault/1 -> rff_ctl/4(i_fault)  "i_fault"
  rff_ctl/1(fault_flg) -> fault_flg/1  "fault_flg"
  rff_ctl/2(ff_count) -> ff_count/1  "ff_count"

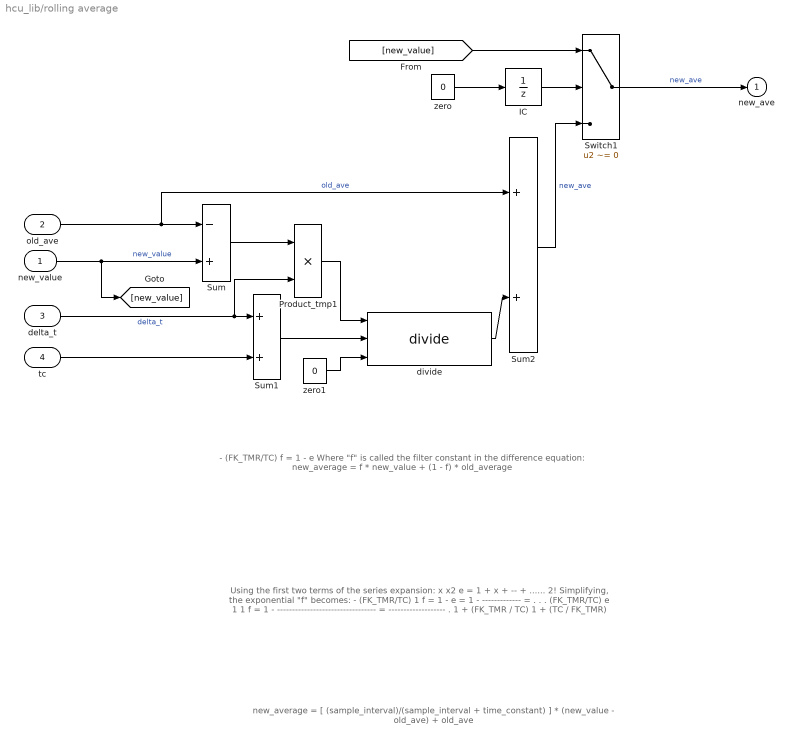
== system hcu_lib/rolling average ==
  note: Using the first two terms of the series expansion:
      |
      |                     x                     x2
      |                                e   =  1  +  x  +  --  + ......
      |                                           2!
      |
      |       Simplifying, the exponential "f" becomes:
      |
      |                  - (FK_TMR/TC)              1
      |           f  =  1  -  e                    =  1  -  -------------  =  . . .
      |                                                    (FK_TMR/TC)
      |                           e
      |
      |                              1                      1
      |          f  =  1  -  ---------------------------------  =    ------------------- .
      |                                  1 + (FK_TMR / TC)       1 + (TC / FK_TMR)
  note: new_average = [ (sample_interval)/(sample_interval + time_constant) ] * (new_value - old_ave) + old_ave
  note: - (FK_TMR/TC)
      |                                    f  =  1  -  e
      |
      |       Where "f" is called the filter constant in the difference equation:
      |
      |                    new_average = f * new_value + (1 - f) * old_average
  new_value : Inport  OutDataType=sfix(16)  OutScaling=2^0
  old_ave : Inport  Port=2  OutDataType=sfix(16)  OutScaling=2^0
  delta_t : Inport  Port=3  OutDataType=sfix(16)  OutScaling=2^0
  tc : Inport  Port=4  OutDataType=sfix(16)  OutScaling=2^0
  IC : UnitDelay  Tag=struct('comment',struct('text','','placement',1),'logdata',struct('maxnumvals',inf,'plotchannels',[],'stepsize',0,'downsampling',1,'loggingmode',3,'channels',1),'output',struct('width',1,'name','$S_$B','unit','','type','Int16','offset',0,'max',NaN,'min',NaN,'freeze',1,'lsb',1,'arb',0,'class','default','address','','description','','autoscalingmode',1,'lowerheadroom',1,'upperheadroom',1,'headroomunit','bit','checkmin',0,'checkmax',0,'show',0,'initial','2'),'state',0,'dt','-1','date',731455.586925799)  X0=1  SampleTime=-1
  Product_tmp1 : Product  Tag=struct('comment',struct('text','','placement',1),'logdata',struct('maxnumvals',inf,'plotchannels',[],'stepsize',0,'downsampling',1,'loggingmode',3,'channels',1),'output',struct('width',1,'name','$S_$B','unit','','type','Int32Bin15','offset',0,'max',65535,'min',-65536,'freeze',1,'lsb',2^-15,'arb',0,'class','default','address','','description','','autoscalingmode',1,'lowerheadroom',1,'upperheadroom',1,'headroomunit','bit','checkmin',0,'checkmax',0,'show',0),'inputs','**','exceptionhandling',1,'date',731455.58640515)  Inputs=**  OutDataType=sfix(16)  OutScaling=2^0  SaturateOnIntegerOverflow=on  RndMeth=Zero  InputSameDT=on  OutDataTypeStr=Inherit: Same as first input
  Sum : Sum  Tag=struct('comment',struct('text','','placement',1),'logdata',struct('maxnumvals',inf,'plotchannels',[],'stepsize',0,'downsampling',1,'loggingmode',3,'channels',1),'output',struct('width',1,'name','$S_$B','unit','','type','Int32Bin15','offset',0,'max',65535,'min',-65536,'freeze',1,'lsb',2^-15,'arb',0,'class','default','address','','description','','autoscalingmode',1,'lowerheadroom',1,'upperheadroom',1,'headroomunit','bit','checkmin',0,'checkmax',0,'show',0),'inputs','-+','date',731455.586330463)  Inputs=-+  OutDataType=sfix(16)  OutScaling=2^0  SaturateOnIntegerOverflow=on  InputSameDT=on  OutDataTypeStr=Inherit: Same as first input
  Sum1 : Sum  Tag=struct('comment',struct('text','','placement',1),'logdata',struct('maxnumvals',inf,'plotchannels',[],'stepsize',0,'downsampling',1,'loggingmode',3,'channels',1),'output',struct('width',1,'name','$S_$B','unit','','type','Int32Bin15','offset',0,'max',65535,'min',-65536,'freeze',1,'lsb',2^-15,'arb',0,'class','default','address','','description','','autoscalingmode',1,'lowerheadroom',1,'upperheadroom',1,'headroomunit','bit','checkmin',0,'checkmax',0,'show',0),'inputs','++','date',731455.58628235)  OutDataType=sfix(16)  OutScaling=2^0  SaturateOnIntegerOverflow=on  InputSameDT=on  OutDataTypeStr=Inherit: Same as first input
  Sum2 : Sum  Tag=struct('comment',struct('text','','placement',1),'logdata',struct('maxnumvals',inf,'plotchannels',[],'stepsize',0,'downsampling',1,'loggingmode',3,'channels',1),'output',struct('width',1,'name','$S_$B','unit','','type','Int32Bin15','offset',0,'max',65535,'min',-65536,'freeze',1,'lsb',2^-15,'arb',0,'class','default','address','','description','','autoscalingmode',1,'lowerheadroom',1,'upperheadroom',1,'headroomunit','bit','checkmin',0,'checkmax',0,'show',0),'inputs','++','date',731455.586506424)  OutDataType=sfix(16)  OutScaling=2^0  SaturateOnIntegerOverflow=on  InputSameDT=on  OutDataTypeStr=Inherit: Same as first input
  Switch1 : Switch  Tag=struct('comment',struct('text','','placement',1),'logdata',struct('maxnumvals',inf,'plotchannels',[],'stepsize',0,'downsampling',1,'loggingmode',3,'channels',1),'output',struct('width',1,'name','$S_$B','unit','','type','Int32Bin15','offset',0,'max',65535,'min',-65536,'freeze',1,'lsb',2^-15,'arb',0,'class','default','address','','description','','autoscalingmode',1,'lowerheadroom',1,'upperheadroom',1,'headroomunit','bit','checkmin',0,'checkmax',0,'show',0),'threshold',struct('width',1,'name','$S_$B_threshold','unit','','type','Int16','offset',0,'max',NaN,'min',NaN,'freeze',1,'lsb',1,'arb',0,'class','default','address','','description','','value','1','scalar',0),'date',731455.58657044)  Criteria=u2 ~= 0  Threshold=0.5
  divide : hcu_lib/divide  SystemSampleTime=-1
  zero : Constant  Tag=struct('comment',struct('text','','placement',1),'output',struct('width',1,'name','$S_$B','unit','','type','Int16','offset',0,'max',NaN,'min',NaN,'freeze',1,'lsb',1,'arb',0,'class','default','address','','description','','value','0','tolerance',1,'show',0),'date',731455.58675544)  Value=0  OutDataTypeMode=boolean  OutDataType=sfix(16)  OutScaling=2^0  OutDataTypeStr=boolean
  zero1 : Constant  Tag=struct('comment',struct('text','','placement',1),'output',struct('width',1,'name','$S_$B','unit','','type','Int16','offset',0,'max',NaN,'min',NaN,'freeze',1,'lsb',1,'arb',0,'class','default','address','','description','','value','0','tolerance',1,'show',0),'date',731455.58675544)  Value=0  OutDataTypeMode=single  OutDataType=sfix(16)  OutScaling=2^0  OutDataTypeStr=single
  new_ave : Outport  OutDataType=sfix(16)  OutScaling=2^0
  wires:
  old_ave/1 -> Sum/1, Sum2/1  "old_ave"
  new_value/1 -> [new_value], Sum/2  "new_value"
  delta_t/1 -> Sum1/1, Product_tmp1/2  "delta_t"
  tc/1 -> Sum1/2
  divide/1 -> Sum2/2
  Sum/1 -> Product_tmp1/1
  zero/1 -> IC/1
  IC/1 -> Switch1/2
  Sum2/1 -> Switch1/3  "new_ave"
  Switch1/1 -> new_ave/1  "new_ave"
  [new_value] -> Switch1/1
  Product_tmp1/1 -> divide/1
  Sum1/1 -> divide/2
  zero1/1 -> divide/3

== system hcu_lib/rpm2radps ==
  u : Inport  OutDataType=sfix(16)  OutScaling=2^0
  Gain : Gain  Gain=RPM2RADPS  ParameterDataType=sfix(16)  ParameterScaling=2^0  OutDataType=sfix(16)  OutScaling=2^0
  y : Outport  OutDataType=sfix(16)  OutScaling=2^0
  wires:
  Gain/1 -> y/1  "y"
  u/1 -> Gain/1  "u"

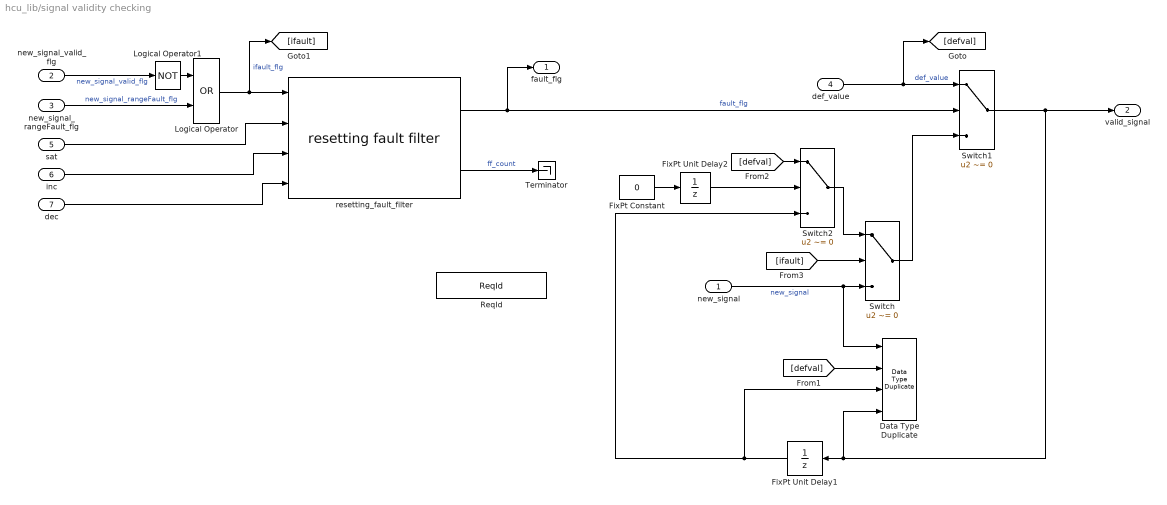
== system hcu_lib/signal validity checking ==
  new_signal : Inport  OutDataType=sfix(16)  OutScaling=2^0
  new_signal_valid_flg : Inport  Port=2  OutDataType=sfix(16)  OutScaling=2^0
  new_signal_rangeFault_flg : Inport  Port=3  OutDataType=sfix(16)  OutScaling=2^0
  def_value : Inport  Port=4  OutDataType=sfix(16)  OutScaling=2^0
  sat : Inport  Port=5  OutDataType=sfix(16)  OutScaling=2^0
  inc : Inport  Port=6  OutDataType=sfix(16)  OutScaling=2^0
  dec : Inport  Port=7  OutDataType=sfix(16)  OutScaling=2^0
  Data Type Duplicate : simulink/Signal Attributes/Data Type Duplicate  NumInputPorts=4
  FixPt Constant : Constant  DisableCoverage=on  Value=0  OutDataTypeMode=Specify via dialog  OutDataType=fixdt(0,8,0)  ConRadixGroup=Best Precision: Vector-wise  OutDataTypeStr=fixdt(0,8,0)
  FixPt Unit Delay1 : UnitDelay  DisableCoverage=on  SampleTime=-1
  FixPt Unit Delay2 : UnitDelay  DisableCoverage=on  X0=1  SampleTime=-1
  Logical Operator : Logic  Tag=struct('inputs','2','comment',struct('text','','placement',1),'logdata',struct('maxnumvals',inf,'plotchannels',[],'stepsize',0,'downsampling',1,'loggingmode',3,'channels',1),'operator','OR','output',struct('class','default','type','Bool8','description','','address','','unit','','name','$S_$B'),'date',731430.467498704)  Operator=OR
  Logical Operator1 : Logic  Tag=struct('inputs','1','comment',struct('text','','placement',1),'logdata',struct('maxnumvals',inf,'plotchannels',[],'stepsize',0,'downsampling',1,'loggingmode',3,'channels',1),'operator','NOT','output',struct('class','default','type','Bool8','description','','address','','unit','','name','$S_$B'),'date',731430.46749816)  Operator=NOT  Inputs=1
  ReqId : hcu_lib/ReqId  SystemSampleTime=-1  req_str=HCU_009
  Switch : Switch  Criteria=u2 ~= 0  OutDataType=fixdt(1, 16)  OutScaling=2^0
  Switch1 : Switch  Criteria=u2 ~= 0  OutDataType=fixdt(1, 16)  OutScaling=2^0
  Switch2 : Switch  Criteria=u2 ~= 0  OutDataType=fixdt(1, 16)  OutScaling=2^0
  Terminator : Terminator
  resetting_fault_filter : hcu_lib/resetting fault filter  SystemSampleTime=-1
  fault_flg : Outport  OutDataType=sfix(16)  OutScaling=2^0
  valid_signal : Outport  Port=2  OutDataType=sfix(16)  OutScaling=2^0
  wires:
  Logical Operator/1 -> resetting_fault_filter/1, [ifault]  "ifault_flg"
  resetting_fault_filter/2 -> Terminator/1  "ff_count"
  resetting_fault_filter/1 -> fault_flg/1, Switch1/2  "fault_flg"
  def_value/1 -> [defval], Switch1/1  "def_value"
  Logical Operator1/1 -> Logical Operator/1
  new_signal/1 -> Switch/3, Data Type Duplicate/1  "new_signal"
  new_signal_valid_flg/1 -> Logical Operator1/1  "new_signal_valid_flg"
  new_signal_rangeFault_flg/1 -> Logical Operator/2  "new_signal_rangeFault_flg"
  sat/1 -> resetting_fault_filter/2
  inc/1 -> resetting_fault_filter/3
  dec/1 -> resetting_fault_filter/4
  Switch/1 -> Switch1/3
  FixPt Constant/1 -> FixPt Unit Delay2/1
  FixPt Unit Delay2/1 -> Switch2/2
  [defval] -> Switch2/1
  Switch2/1 -> Switch/1
  Switch1/1 -> valid_signal/1, FixPt Unit Delay1/1, Data Type Duplicate/4
  [ifault] -> Switch/2
  FixPt Unit Delay1/1 -> Switch2/3, Data Type Duplicate/3
  [defval] -> Data Type Duplicate/2

== system hcu_lib/unit_conversion ==
  input_signal : Inport  OutDataType=sfix(16)  OutScaling=2^0
  signal_gain : Inport  Port=2  OutDataType=sfix(16)  OutScaling=2^0
  signal_offset : Inport  Port=3  OutDataType=sfix(16)  OutScaling=2^0
  Product : Product  OutDataType=sfix(16)  OutScaling=2^0  RndMeth=Zero
  Sum : Sum  OutDataType=sfix(16)  OutScaling=2^0
  output_signal : Outport  OutDataType=sfix(16)  OutScaling=2^0
  wires:
  signal_offset/1 -> Sum/2  "signal_offset"
  Sum/1 -> output_signal/1  "output_signal"
  Product/1 -> Sum/1
  input_signal/1 -> Product/2  "input_signal"
  signal_gain/1 -> Product/1  "signal_gain"

== system hcu_lib/xx2kxx ==
  u : Inport  OutDataType=sfix(16)  OutScaling=2^0
  Gain : Gain  Gain=0.001  ParameterDataType=sfix(16)  ParameterScaling=2^0  OutDataType=sfix(16)  OutScaling=2^0
  y : Outport  OutDataType=sfix(16)  OutScaling=2^0
  wires:
  u/1 -> Gain/1  "u"
  Gain/1 -> y/1  "y"

== stateflow chart latching hold fault filter/lhff_ctl ==
  (default) -> (junction 3)
  (junction 7) -> (junction 8) [order 2] : {count-=dec;}
  (junction 3) -> (junction 9) [order 1] : [i_fault]
      | {count+=inc;}
  (junction 4) -> (junction 5) [order 1] : [count>=sat]
      | {count=sat;
      |  fault_flg=1;}
  (junction 4) -> (junction 5) [order 2] : [count<=0]
      | {count=0;}
  (junction 4) -> (junction 5) [order 3]
  (junction 5) -> (junction 6) : {ff_count = count;}
  (junction 7) -> (junction 8) [order 1] : [hold]
  (junction 3) -> (junction 7) [order 2]
  (junction 8) -> (junction 9)
  (junction 9) -> (junction 4)
  data: sat input uint8; inc input uint8; dec input uint8; i_fault input boolean; fault_flg output boolean; ff_count output uint8; count local int16; hold input boolean

== stateflow chart resetting fault filter/rff_ctl ==
  (default) -> (junction 31)
  (junction 31) -> (junction 35) [order 2] : {count-=dec;}
  (junction 31) -> (junction 35) [order 1] : [i_fault]
      | {count+=inc;}
  (junction 32) -> (junction 33) [order 1] : [count>=sat]
      | {count=sat;
      | fault_flg=1;}
  (junction 32) -> (junction 33) [order 2] : [count<=0]
      | {count=0;
      | fault_flg=0;}
  (junction 32) -> (junction 33) [order 3]
  (junction 33) -> (junction 34) : {ff_count = count;}
  (junction 35) -> (junction 32)
  data: sat input uint8; inc input uint8; dec input uint8; i_fault input boolean; fault_flg output boolean =0; ff_count output uint8; count local int16

== stateflow chart latching fault filter/lff_ctl ==
  (default) -> (junction 53)
  (junction 53) -> (junction 57) [order 2] : {count-=dec;}
  (junction 53) -> (junction 57) [order 1] : [i_fault]
      | {count+=inc;}
  (junction 54) -> (junction 55) [order 1] : [count>=sat]
      | {count=sat;
      | fault_flg=1;}
  (junction 54) -> (junction 55) [order 2] : [count<=0]
      | {count=0;}
  (junction 54) -> (junction 55) [order 3]
  (junction 55) -> (junction 56) : {ff_count = count;}
  (junction 57) -> (junction 54)
  data: sat input uint8; inc input uint8; dec input uint8; i_fault input boolean; fault_flg output boolean =0; ff_count output uint8; count local int16 =0
